simulink model "OFDM_QAM_512"  (R2017a)
settings: Solver=VariableStepAuto  StartTime=0.0  StopTime=inf  RelTol=1e-3
model workspace (MAT data in the model file):
  M = 16
libraries: dspxfrm3 x3, dspindex x2, commdigbbndam3 x2, commchan3 x1, commsink2 x1, commrandsrc2 x1
settings Model: Creator=Sommc  LastModifiedBy=romainsercer

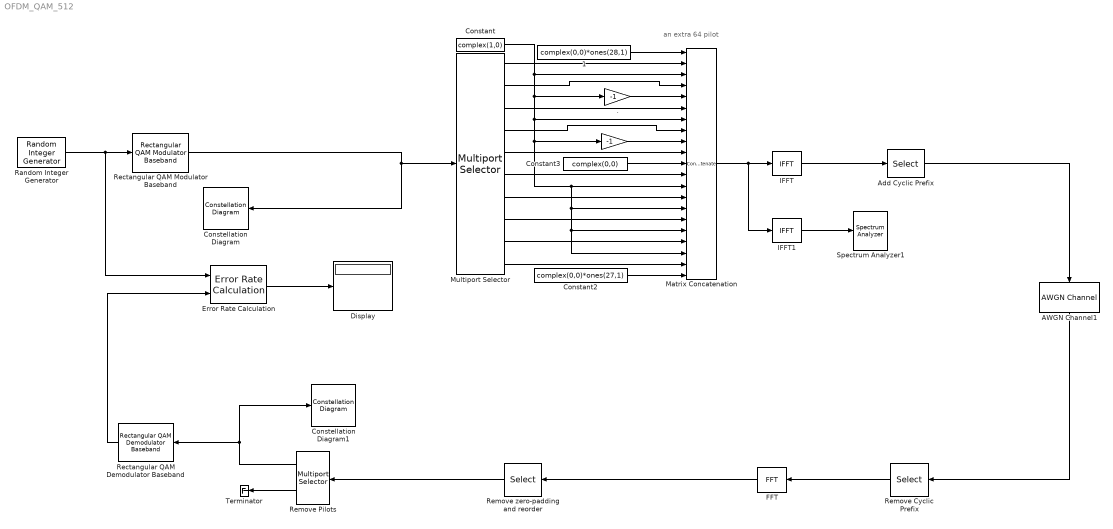
== system OFDM_QAM_512 ==
  note: an extra 64 pilot
  " " : Gain  Gain=-1
  " 1" : Constant  Value=complex(0,0)*ones(28,1)
  . : Gain  Gain=-1
  AWGN Channel1 : commchan3/AWGN Channel  InputProcessing=Inherited (this choice will be removed - see release notes)  seed=34  noiseMode="Signal to noise ratio  (SNR)"  EbNodB=10  EsNodB=40  SNRdB=20  bitsPerSym=2  Ps=0.01  Tsym=4e-6/80  variance=1
  Add Cyclic Prefix : Selector  InputPortWidth=512  IndexOptions=Index vector (dialog)  Indices=[497:512 1:512]  OutputSizes=[(-2)]
  Constant : Constant  Value=complex(1,0)
  Constant2 : Constant  Value=complex(0,0)*ones(27,1)
  Constant3 : Constant  Value=complex(0,0)
  Constellation Diagram : ConstellationDiagram
  Constellation Diagram1 : ConstellationDiagram
  Display : Display
  Error Rate Calculation : commsink2/Error Rate Calculation  N=0  st_delay=0  cp_mode=Entire frame  subframe=[]  PMode=Port  WsName=ErrorVec  RsMode2=off  stop=off  numErr=100  maxBits=1e6
  FFT : dspxfrm3/FFT  FFTImplementation=Auto  CompMethod=Table lookup  TableOpt=HYBRID  TableOptActive=Speed  BitRevOrder=off  Normalize=off  InheritFFTLength=off  FFTLength=512  WrapInput=on  roundingMode=Floor  overflowMode=off  firstCoeffDataTypeStr=Inherit: Same word length as input  firstCoeffLastDataTypeStr=Inherit: Same word length as input  outputMin=[]  outputMax=[]
  IFFT : dspxfrm3/IFFT  FFTImplementation=Auto  CompMethod=Table lookup  TableOpt=HYBRID  TableOptActive=Speed  BitRevOrder=off  cs_in=off  Normalize=on  InheritFFTLength=on  FFTLength=512  WrapInput=off  mode=Complex  outSamplingMode=Frame based  roundingMode=Floor  overflowMode=off  firstCoeffDataTypeStr=Inherit: Same word length as input  firstCoeffLastDataTypeStr=Inherit: Same word length as input  outputMin=[]  outputMax=[]
      settings: SourceProductName=DSP System Toolbox
  IFFT1 : dspxfrm3/IFFT  FFTImplementation=Auto  CompMethod=Table lookup  TableOpt=HYBRID  TableOptActive=Speed  BitRevOrder=off  cs_in=on  Normalize=on  InheritFFTLength=on  FFTLength=512  WrapInput=on  mode=Complex  outSamplingMode=Frame based  roundingMode=Floor  overflowMode=off  firstCoeffDataTypeStr=Inherit: Same word length as input  firstCoeffLastDataTypeStr=Inherit: Same word length as input  outputMin=[]  outputMax=[]
      settings: SourceProductName=DSP System Toolbox
  Matrix Concatenation : Concatenate  NumInputs=21  Mode=Multidimensional array
  Multiport Selector : dspindex/Multiport Selector  rowsOrCols=Rows  idxCellArray={1:32, 33:80, 81:128, 129:176, 177:224, 225:272, 273:320, 321:368, 369:416, 417:448}  idxErrMode=Clip Index
  Random Integer Generator : commrandsrc2/Random Integer Generator  mul=M  seed=37  Ts=1/7.5e6  frameBased=on  sampPerFrame=448  orient=off  outDataType=double
  Rectangular QAM Demodulator Baseband : commdigbbndam3/Rectangular QAM Demodulator Baseband  M=M  OutType=Integer  DecType=Hard decision  VarSource=Dialog  Variance=1  Dec=Gray  Mapping=[0:15]  PowType=Min. distance between symbols  MinDist=1  AvgPow=1  PeakPow=1  Ph=0  outDtype1=Inherit via internal rule  outDtype2=Inherit via internal rule  derotateFactorWordLen=16  derotateFactorDataTypeStr=Inherit: Same word length as input  derotateFactorLastDataTypeStr=Inherit: Same word length as input  denormFactorWordLen=16  denormFactorDataTypeStr=Inherit: Same word length as input  denormFactorLastDataTypeStr=Inherit: Same word length as input  prodOutWordLen=32  prodOutOverflowMode=Wrap  prodOutRoundingMode=Floor  prodOutOvFlMode=off  prodOutOvFlModeLastStrValue=off  sumWordLen=32
  Rectangular QAM Modulator Baseband : commdigbbndam3/Rectangular QAM Modulator Baseband  M=M  InType=Integer  Enc=Gray  Mapping=[0:15]  PowType=Min. distance between symbols  MinDist=1  AvgPow=1  PeakPow=1  Ph=0  outDtype=double  outWordLen=16  outUDDataType=sfix(16)  outFracLenMode=Best precision  outFracLen=15  outDataTypeStr=double  outLastDataTypeStr=double
  Remove zero-padding and reorder : Selector  InputPortWidth=512  IndexOptions=Index vector (dialog)  Indices=[29:256 258:485]  OutputSizes=[(-2)]
  Remove Pilots : dspindex/Multiport Selector  rowsOrCols=Rows  idxCellArray={[1:32 34:81 83:130 132:179 181:276 278:325 327:374 376:423 425:456 ],[33 82 131 180 277 326 375 424]}  idxErrMode=Clip Index
  Remove Cyclic Prefix : Selector  InputPortWidth=528  IndexOptions=Index vector (dialog)  Indices=[17:528]  OutputSizes=[(-2)]
  Spectrum Analyzer1 : SpectrumAnalyzer
  Terminator : Terminator
  wires:
  Random Integer Generator/1 -> Error Rate Calculation/1, Rectangular QAM Modulator Baseband/1
  Matrix Concatenation/1 -> IFFT1/1, IFFT/1
  IFFT/1 -> Add Cyclic Prefix/1
  Constant3/1 -> Matrix Concatenation/11
  " "/1 -> Matrix Concatenation/9
  ./1 -> Matrix Concatenation/5
  Constant2/1 -> Matrix Concatenation/21
  " 1"/1 -> Matrix Concatenation/1
  Constant/1 -> ./1, Matrix Concatenation/17, Matrix Concatenation/19, Matrix Concatenation/15, Matrix Concatenation/13, " "/1, Matrix Concatenation/7, Matrix Concatenation/3
  Multiport Selector/10 -> Matrix Concatenation/20
  Multiport Selector/1 -> Matrix Concatenation/2
  Multiport Selector/2 -> Matrix Concatenation/4
  Multiport Selector/3 -> Matrix Concatenation/6
  Multiport Selector/4 -> Matrix Concatenation/8
  Multiport Selector/5 -> Matrix Concatenation/10
  Multiport Selector/6 -> Matrix Concatenation/12
  Multiport Selector/7 -> Matrix Concatenation/14
  Multiport Selector/8 -> Matrix Concatenation/16
  Multiport Selector/9 -> Matrix Concatenation/18
  Rectangular QAM Modulator Baseband/1 -> Constellation Diagram/1, Multiport Selector/1
  Remove Pilots/2 -> Terminator/1
  Remove Pilots/1 -> Constellation Diagram1/1, Rectangular QAM Demodulator Baseband/1
  Remove zero-padding and reorder/1 -> Remove Pilots/1
  FFT/1 -> Remove zero-padding and reorder/1
  Rectangular QAM Demodulator Baseband/1 -> Error Rate Calculation/2
  Error Rate Calculation/1 -> Display/1
  Remove Cyclic Prefix/1 -> FFT/1
  Add Cyclic Prefix/1 -> AWGN Channel1/1
  AWGN Channel1/1 -> Remove Cyclic Prefix/1
  IFFT1/1 -> Spectrum Analyzer1/1
